simulink model "SLIP_ratio_slip_angle"  (R2015a)
settings: Solver=ode45  StartTime=0.0  StopTime=10.0  RelTol=1e-3
settings Model: Creator=BML  LastModifiedBy=BML

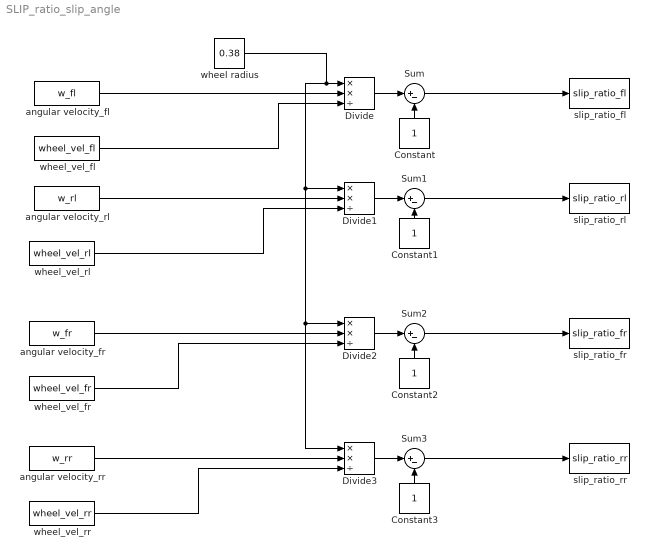
== system SLIP_ratio_slip_angle ==
  Constant{,1..3} (4 alike) : Constant
  Divide{,1..3} (4 alike) : Product  Inputs=**/
  Sum{,1..3} (4 alike) : Sum  Inputs=|+-
  angular velocity_fl : FromWorkspace  VariableName=w_fl  SampleTime=0
  angular velocity_fr : FromWorkspace  VariableName=w_fr  SampleTime=0
  angular velocity_rl : FromWorkspace  VariableName=w_rl  SampleTime=0
  angular velocity_rr : FromWorkspace  VariableName=w_rr  SampleTime=0
  slip_ratio_fl : ToWorkspace  VariableName=slip_ratio_fl  SaveFormat=Timeseries  SampleTime=-1
  slip_ratio_fr : ToWorkspace  VariableName=slip_ratio_fr  SaveFormat=Timeseries  SampleTime=-1
  slip_ratio_rl : ToWorkspace  VariableName=slip_ratio_rl  SaveFormat=Timeseries  SampleTime=-1
  slip_ratio_rr : ToWorkspace  VariableName=slip_ratio_rr  SaveFormat=Timeseries  SampleTime=-1
  wheel radius : Constant  Value=0.38
  wheel_vel_fl : FromWorkspace  VariableName=wheel_vel_fl  SampleTime=0
  wheel_vel_fr : FromWorkspace  VariableName=wheel_vel_fr  SampleTime=0
  wheel_vel_rl : FromWorkspace  VariableName=wheel_vel_rl  SampleTime=0
  wheel_vel_rr : FromWorkspace  VariableName=wheel_vel_rr  SampleTime=0
  wires:
  angular velocity_fl/1 -> Divide/2
  wheel_vel_fl/1 -> Divide/3
  Divide/1 -> Sum/1
  Sum/1 -> slip_ratio_fl/1
  Constant/1 -> Sum/2
  angular velocity_rl/1 -> Divide1/2
  wheel_vel_rl/1 -> Divide1/3
  Divide1/1 -> Sum1/1
  Constant1/1 -> Sum1/2
  Sum1/1 -> slip_ratio_rl/1
  angular velocity_fr/1 -> Divide2/2
  wheel_vel_fr/1 -> Divide2/3
  Divide2/1 -> Sum2/1
  Constant2/1 -> Sum2/2
  Sum2/1 -> slip_ratio_fr/1
  wheel radius/1 -> Divide3/1, Divide2/1, Divide1/1, Divide/1
  angular velocity_rr/1 -> Divide3/2
  wheel_vel_rr/1 -> Divide3/3
  Divide3/1 -> Sum3/1
  Constant3/1 -> Sum3/2
  Sum3/1 -> slip_ratio_rr/1
